simulink model "user_specified_execution_order"  (Simulink 6.6)
settings: Solver=FixedStepDiscrete  StartTime=0.0  StopTime=10.0  FixedStep=1  RelTol=1e-3
settings Model: Creator=vBuskirk  LastModifiedBy=vBuskirk

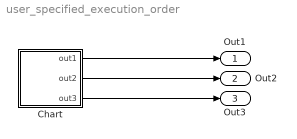
== system user_specified_execution_order ==
  Chart : Stateflow chart
  Out1 : Outport
  Out2 : Outport  Port=2
  Out3 : Outport  Port=3
  wires:
  Chart/1(out1) -> Out1/1
  Chart/2(out2) -> Out2/1
  Chart/3(out3) -> Out3/1

== stateflow chart Chart ==
  state M1 [parallel]
    settings: executionOrder=1
    state s1
      en:out1=1;
    state s2
      en:out1=2;
    state s3
      en:out1=3;
    (default) -> M1.s1
    M1.s1 -> M1.s2 [order 2]
    M1.s1 -> M1.s3 [order 1]
  state M2 [parallel]
    settings: executionOrder=2
    state s1 [parallel]
      en:out2=1;
      settings: executionOrder=2
    state s2 [parallel]
      en:out2=2;
      settings: executionOrder=3
    state s3 [parallel]
      en:out2=3;
      settings: executionOrder=1
  state M3 [parallel]
    settings: executionOrder=3
    state s1
    state s2
    state s3
    (default) -> M3.s1
    M3.s1 -> M3.s2 [order 2] : / out3=2;
    M3.s1 -> M3.s3 [order 1] : / out3=3;
  data: out1 output double =-100; out2 output double =-200; out3 output double =-300
